simulink model "Exmaple"  (R2017b)
settings: Solver=VariableStepAuto  StartTime=0.0  StopTime=inf  RelTol=1e-3
libraries: Project1_Library x4, realtime_pacer_lib x1
settings Model: Creator=hattanbadyah  LastModifiedBy=hattanbadyah

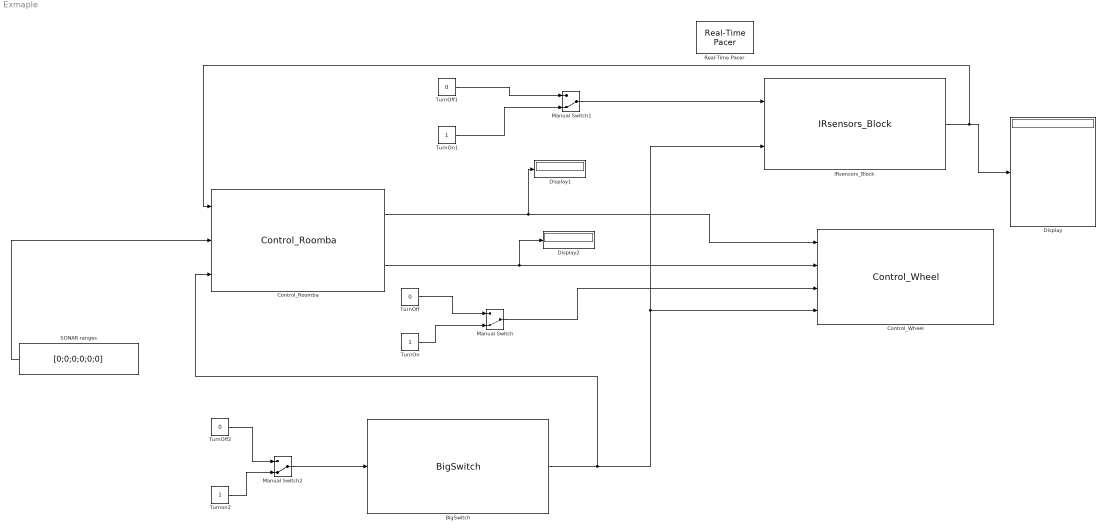
== system Exmaple ==
  BigSwitch : Project1_Library/BigSwitch
  Control_Roomba : Project1_Library/Control_Roomba  SystemSampleTime=-1
  Control_Wheel : Project1_Library/Control_Wheel
  Display : Display
  Display1 : Display
  Display2 : Display
  IRsensors_Block : Project1_Library/IRsensors_Block
  Manual Switch : ManualSwitch  CurrentSetting=0
  Manual Switch1 : ManualSwitch  CurrentSetting=0
  Manual Switch2 : ManualSwitch  CurrentSetting=0
  Real-Time Pacer : realtime_pacer_lib/Real-Time Pacer  simTimePerRealTime=1
  SONAR ranges : Constant  Value=[0;0;0;0;0;0]
  TurnOff : Constant  Value=0
  TurnOff1 : Constant  Value=0
  TurnOff2 : Constant  Value=0
  TurnOn : Constant
  TurnOn1 : Constant
  Turnon2 : Constant
  wires:
  BigSwitch/1 -> Control_Roomba/3, IRsensors_Block/2, Control_Wheel/4
  Control_Roomba/1 -> Display1/1, Control_Wheel/1
  Control_Roomba/2 -> Display2/1, Control_Wheel/2
  TurnOff/1 -> Manual Switch/1
  TurnOn/1 -> Manual Switch/2
  Manual Switch/1 -> Control_Wheel/3
  Manual Switch1/1 -> IRsensors_Block/1
  TurnOff1/1 -> Manual Switch1/1
  TurnOn1/1 -> Manual Switch1/2
  IRsensors_Block/1 -> Control_Roomba/1, Display/1
  Manual Switch2/1 -> BigSwitch/1
  TurnOff2/1 -> Manual Switch2/1
  Turnon2/1 -> Manual Switch2/2
  SONAR ranges/1 -> Control_Roomba/2
